simulink model "gm_fft_overlap_tomori"  (R2023b)
settings: Solver=VariableStepAuto  StartTime=0.0  StopTime=inf  RelTol=1e-3
InitFcn:
  | fftparrallelout
  | load('dataram.mat')
  | s= fi(exp(-1j*2*pi.*(0:63)/64),1,16,15);
  | fixed_point = fixdt(1,27,20);
  | fixed_pointu = fixdt(0,29,20);
  | fixed = fixdt(1,22,15);
  | const = fixdt(1,18,17);
  | addConst = fixdt(1,18,16);
  | f =10.4e6;
  | f1=45e6;
  | alpha1 =5;
  | beta1 = 0.00001 ;
  | beta2 = 0.99999 ;
  | beta3 = 23;
undefined symbols (not defined in the file or in its folder): j
libraries: dspxfrm3 x11, commrflib2 x4
(part 6 of 10)

== system gm_fft_overlap_tomori/16//32 and test junk/32/FFT32/FFT16/FFT8 ==
  In1 : Inport
  In2 : Inport  Port=2
  In3 : Inport  Port=3
  In4 : Inport  Port=4
  In5 : Inport  Port=5
  In6 : Inport  Port=6
  In7 : Inport  Port=7
  In8 : Inport  Port=8
  Add{,2,4,6,8,10,12,14,16,18,20,22} (12 alike) : Sum  OutDataTypeStr=fixed  RndMeth=Round
  Add{1,3,5,7,9,11,13,15,17,19,21,23} (12 alike) : Sum  Inputs=+-  OutDataTypeStr=fixed  RndMeth=Round
  Delay{,1,4..9,12..13,16..23} (18 alike) : Delay  DelayLength=1
  Delay{2..3,10..11,14..15} (6 alike) : Delay  DelayLength=3
  multByExp(-j*Pi/4) : Subsystem
  multByExp(-j*Pi/4)1 : Subsystem
  multByMinusJ : Subsystem
  multByMinusJ1 : Subsystem
  multByMinusJ2 : Subsystem
  multByMinusJ3 : Subsystem
  x0 : Outport
  x1 : Outport  Port=2  VectorParamsAs1DForOutWhenUnconnected=off
  x2 : Outport  Port=3  VectorParamsAs1DForOutWhenUnconnected=off
  x3 : Outport  Port=4  VectorParamsAs1DForOutWhenUnconnected=off
  x4 : Outport  Port=5  VectorParamsAs1DForOutWhenUnconnected=off
  x5 : Outport  Port=6  VectorParamsAs1DForOutWhenUnconnected=off
  x6 : Outport  Port=7  VectorParamsAs1DForOutWhenUnconnected=off
  x7 : Outport  Port=8  VectorParamsAs1DForOutWhenUnconnected=off
  wires:
  Delay17/1 -> Add21/2, Add20/2
  Delay15/1 -> Add21/1, Add20/1
  Delay23/1 -> x7/1
  Delay22/1 -> x3/1
  Delay21/1 -> x5/1
  Delay20/1 -> x1/1
  multByExp(-j*Pi/4)1/1(Out1) -> multByMinusJ3/1(In1)
  multByExp(-j*Pi/4)/1(Out1) -> Delay16/1
  multByMinusJ3/1(Out1) -> Delay17/1
  Delay16/1 -> Add18/2, Add19/2
  Delay14/1 -> Add19/1, Add18/1
  Add21/1 -> Delay23/1
  Add20/1 -> Delay22/1
  Add19/1 -> Delay21/1
  Add18/1 -> Delay20/1
  Delay19/1 -> x6/1
  Delay18/1 -> x2/1
  Delay11/1 -> Add12/2, Add13/2
  multByMinusJ2/1(Out1) -> Delay11/1
  Add13/1 -> Delay19/1
  Add12/1 -> Delay18/1
  Delay3/1 -> Add12/1, Add13/1
  Add17/1 -> multByExp(-j*Pi/4)1/1(In1)
  Add16/1 -> multByExp(-j*Pi/4)/1(In1)
  Delay9/1 -> Add16/2, Add17/2
  Delay5/1 -> Add16/1, Add17/1
  multByMinusJ1/1(Out1) -> Delay9/1
  multByMinusJ/1(Out1) -> Delay7/1
  Add15/1 -> Delay15/1
  Add14/1 -> Delay14/1
  Delay7/1 -> Add15/2, Add14/2
  Delay1/1 -> Add15/1, Add14/1
  Delay13/1 -> x4/1
  Delay12/1 -> x0/1
  Add23/1 -> Delay13/1
  Add22/1 -> Delay12/1
  Delay10/1 -> Add22/2, Add23/2
  Delay2/1 -> Add23/1, Add22/1
  Delay6/1 -> Add3/2, Add2/2
  Add11/1 -> multByMinusJ2/1(In1)
  Add10/1 -> Delay10/1
  Delay8/1 -> Add10/2, Add11/2
  Delay4/1 -> Add11/1, Add10/1
  Add9/1 -> multByMinusJ1/1(In1)
  Add8/1 -> Delay8/1
  Add7/1 -> multByMinusJ/1(In1)
  Add6/1 -> Delay6/1
  Add5/1 -> Delay5/1
  Add4/1 -> Delay4/1
  In8/1 -> Add9/2, Add8/2
  In4/1 -> Add8/1, Add9/1
  In6/1 -> Add5/2, Add4/2
  In2/1 -> Add4/1, Add5/1
  In7/1 -> Add7/2, Add6/2
  In3/1 -> Add6/1, Add7/1
  Add3/1 -> Delay3/1
  Add2/1 -> Delay2/1
  Delay/1 -> Add3/1, Add2/1
  Add1/1 -> Delay1/1
  Add/1 -> Delay/1
  In5/1 -> Add1/2, Add/2
  In1/1 -> Add/1, Add1/1

== system gm_fft_overlap_tomori/16//32 and test junk/32/FFT32/FFT16/FFT8_1 ==
  In1 : Inport
  In2 : Inport  Port=2
  In3 : Inport  Port=3
  In4 : Inport  Port=4
  In5 : Inport  Port=5
  In6 : Inport  Port=6
  In7 : Inport  Port=7
  In8 : Inport  Port=8
  Add{,2,4,6,8,10,12,14,16,18,20,22} (12 alike) : Sum  OutDataTypeStr=fixed  RndMeth=Round
  Add{1,3,5,7,9,11,13,15,17,19,21,23} (12 alike) : Sum  Inputs=+-  OutDataTypeStr=fixed  RndMeth=Round
  Delay{,1,4..9,12..13,16..23} (18 alike) : Delay  DelayLength=1
  Delay{2..3,10..11,14..15} (6 alike) : Delay  DelayLength=3
  multByExp(-j*Pi/4) : Subsystem
  multByExp(-j*Pi/4)1 : Subsystem
  multByMinusJ : Subsystem
  multByMinusJ1 : Subsystem
  multByMinusJ2 : Subsystem
  multByMinusJ3 : Subsystem
  x0 : Outport
  x1 : Outport  Port=2  VectorParamsAs1DForOutWhenUnconnected=off
  x2 : Outport  Port=3  VectorParamsAs1DForOutWhenUnconnected=off
  x3 : Outport  Port=4  VectorParamsAs1DForOutWhenUnconnected=off
  x4 : Outport  Port=5  VectorParamsAs1DForOutWhenUnconnected=off
  x5 : Outport  Port=6  VectorParamsAs1DForOutWhenUnconnected=off
  x6 : Outport  Port=7  VectorParamsAs1DForOutWhenUnconnected=off
  x7 : Outport  Port=8  VectorParamsAs1DForOutWhenUnconnected=off
  wires:
  Delay17/1 -> Add21/2, Add20/2
  Delay15/1 -> Add21/1, Add20/1
  Delay23/1 -> x7/1
  Delay22/1 -> x3/1
  Delay21/1 -> x5/1
  Delay20/1 -> x1/1
  multByExp(-j*Pi/4)1/1(Out1) -> multByMinusJ3/1(In1)
  multByExp(-j*Pi/4)/1(Out1) -> Delay16/1
  multByMinusJ3/1(Out1) -> Delay17/1
  Delay16/1 -> Add18/2, Add19/2
  Delay14/1 -> Add19/1, Add18/1
  Add21/1 -> Delay23/1
  Add20/1 -> Delay22/1
  Add19/1 -> Delay21/1
  Add18/1 -> Delay20/1
  Delay19/1 -> x6/1
  Delay18/1 -> x2/1
  Delay11/1 -> Add12/2, Add13/2
  multByMinusJ2/1(Out1) -> Delay11/1
  Add13/1 -> Delay19/1
  Add12/1 -> Delay18/1
  Delay3/1 -> Add12/1, Add13/1
  Add17/1 -> multByExp(-j*Pi/4)1/1(In1)
  Add16/1 -> multByExp(-j*Pi/4)/1(In1)
  Delay9/1 -> Add16/2, Add17/2
  Delay5/1 -> Add16/1, Add17/1
  multByMinusJ1/1(Out1) -> Delay9/1
  multByMinusJ/1(Out1) -> Delay7/1
  Add15/1 -> Delay15/1
  Add14/1 -> Delay14/1
  Delay7/1 -> Add15/2, Add14/2
  Delay1/1 -> Add15/1, Add14/1
  Delay13/1 -> x4/1
  Delay12/1 -> x0/1
  Add23/1 -> Delay13/1
  Add22/1 -> Delay12/1
  Delay10/1 -> Add22/2, Add23/2
  Delay2/1 -> Add23/1, Add22/1
  Delay6/1 -> Add3/2, Add2/2
  Add11/1 -> multByMinusJ2/1(In1)
  Add10/1 -> Delay10/1
  Delay8/1 -> Add10/2, Add11/2
  Delay4/1 -> Add11/1, Add10/1
  Add9/1 -> multByMinusJ1/1(In1)
  Add8/1 -> Delay8/1
  Add7/1 -> multByMinusJ/1(In1)
  Add6/1 -> Delay6/1
  Add5/1 -> Delay5/1
  Add4/1 -> Delay4/1
  In8/1 -> Add9/2, Add8/2
  In4/1 -> Add8/1, Add9/1
  In6/1 -> Add5/2, Add4/2
  In2/1 -> Add4/1, Add5/1
  In7/1 -> Add7/2, Add6/2
  In3/1 -> Add6/1, Add7/1
  Add3/1 -> Delay3/1
  Add2/1 -> Delay2/1
  Delay/1 -> Add3/1, Add2/1
  Add1/1 -> Delay1/1
  Add/1 -> Delay/1
  In5/1 -> Add1/2, Add/2
  In1/1 -> Add/1, Add1/1

== system gm_fft_overlap_tomori/16//32 and test junk/32/FFT32/FFT16/complexmult ==
  x1 : Inport
  In3 : Inport  Port=2
  Add1 : Sum  OutDataTypeStr=fixed  RndMeth=Round
  Add20 : Sum  OutDataTypeStr=fixed  RndMeth=Round
  Add3 : Sum  Inputs=+--  OutDataTypeStr=fixed  AccumDataTypeStr=fixed  RndMeth=Round
  Add4 : Sum  Inputs=+-  OutDataTypeStr=fixed  AccumDataTypeStr=fixed  RndMeth=Round
  Complex to Real-Imag : ComplexToRealImag
  Complex to Real-Imag1 : ComplexToRealImag
  Constant : Constant  Commented=on  Value=1+j  OutDataTypeStr=fixdt(1,22, 15)  SampleTime=2e-8
  Constant1 : Constant  Commented=on  Value=1-j  OutDataTypeStr=fixdt(1,22, 15)  SampleTime=2e-8
  Delay : Delay  DelayLength=3
  Delay1 : Delay  DelayLength=3
  Delay2 : Delay  DelayLength=3
  Display : Display  Commented=on
  Product : Product  OutDataTypeStr=fixed  RndMeth=Round
  Product1 : Product  OutDataTypeStr=fixed  RndMeth=Round
  Product2 : Product  OutDataTypeStr=fixed  RndMeth=Round
  Real-Imag to Complex : RealImagToComplex
  Out1 : Outport
  wires:
  Real-Imag to Complex/1 -> Out1/1
  In3/1 -> Complex to Real-Imag1/1
  x1/1 -> Complex to Real-Imag/1
  Product/1 -> Delay/1
  Product1/1 -> Delay1/1
  Product2/1 -> Delay2/1
  Delay/1 -> Add3/1
  Delay1/1 -> Add4/1, Add3/2
  Delay2/1 -> Add3/3, Add4/2
  Add4/1 -> Real-Imag to Complex/1
  Add3/1 -> Real-Imag to Complex/2
  Add20/1 -> Product/1
  Add1/1 -> Product/2
  Complex to Real-Imag/1 -> Product1/1, Add20/1
  Complex to Real-Imag1/1 -> Product1/2, Add1/1
  Complex to Real-Imag/2 -> Product2/1, Add20/2
  Complex to Real-Imag1/2 -> Product2/2, Add1/2

== system gm_fft_overlap_tomori/16//32 and test junk/32/FFT32/FFT16/complexmult1 ==
  x1 : Inport
  In3 : Inport  Port=2
  Add1 : Sum  OutDataTypeStr=fixed  RndMeth=Round
  Add20 : Sum  OutDataTypeStr=fixed  RndMeth=Round
  Add3 : Sum  Inputs=+--  OutDataTypeStr=fixed  AccumDataTypeStr=fixed  RndMeth=Round
  Add4 : Sum  Inputs=+-  OutDataTypeStr=fixed  AccumDataTypeStr=fixed  RndMeth=Round
  Complex to Real-Imag : ComplexToRealImag
  Complex to Real-Imag1 : ComplexToRealImag
  Constant : Constant  Commented=on  Value=1+j  OutDataTypeStr=fixdt(1,22, 15)  SampleTime=2e-8
  Constant1 : Constant  Commented=on  Value=1-j  OutDataTypeStr=fixdt(1,22, 15)  SampleTime=2e-8
  Delay : Delay  DelayLength=3
  Delay1 : Delay  DelayLength=3
  Delay2 : Delay  DelayLength=3
  Display : Display  Commented=on
  Product : Product  OutDataTypeStr=fixed  RndMeth=Round
  Product1 : Product  OutDataTypeStr=fixed  RndMeth=Round
  Product2 : Product  OutDataTypeStr=fixed  RndMeth=Round
  Real-Imag to Complex : RealImagToComplex
  Out1 : Outport
  wires:
  Complex to Real-Imag1/2 -> Add1/2, Product2/2
  Complex to Real-Imag/2 -> Add20/2, Product2/1
  Complex to Real-Imag1/1 -> Add1/1, Product1/2
  Complex to Real-Imag/1 -> Add20/1, Product1/1
  Add1/1 -> Product/2
  Add20/1 -> Product/1
  Add3/1 -> Real-Imag to Complex/2
  Add4/1 -> Real-Imag to Complex/1
  Delay2/1 -> Add4/2, Add3/3
  Delay1/1 -> Add3/2, Add4/1
  Delay/1 -> Add3/1
  Product2/1 -> Delay2/1
  Product1/1 -> Delay1/1
  Product/1 -> Delay/1
  x1/1 -> Complex to Real-Imag/1
  In3/1 -> Complex to Real-Imag1/1
  Real-Imag to Complex/1 -> Out1/1

== system gm_fft_overlap_tomori/16//32 and test junk/32/FFT32/FFT16/complexmult2 ==
  x1 : Inport
  In3 : Inport  Port=2
  Add1 : Sum  OutDataTypeStr=fixed  RndMeth=Round
  Add20 : Sum  OutDataTypeStr=fixed  RndMeth=Round
  Add3 : Sum  Inputs=+--  OutDataTypeStr=fixed  AccumDataTypeStr=fixed  RndMeth=Round
  Add4 : Sum  Inputs=+-  OutDataTypeStr=fixed  AccumDataTypeStr=fixed  RndMeth=Round
  Complex to Real-Imag : ComplexToRealImag
  Complex to Real-Imag1 : ComplexToRealImag
  Constant : Constant  Commented=on  Value=1+j  OutDataTypeStr=fixdt(1,22, 15)  SampleTime=2e-8
  Constant1 : Constant  Commented=on  Value=1-j  OutDataTypeStr=fixdt(1,22, 15)  SampleTime=2e-8
  Delay : Delay  DelayLength=3
  Delay1 : Delay  DelayLength=3
  Delay2 : Delay  DelayLength=3
  Display : Display  Commented=on
  Product : Product  OutDataTypeStr=fixed  RndMeth=Round
  Product1 : Product  OutDataTypeStr=fixed  RndMeth=Round
  Product2 : Product  OutDataTypeStr=fixed  RndMeth=Round
  Real-Imag to Complex : RealImagToComplex
  Out1 : Outport
  wires:
  Real-Imag to Complex/1 -> Out1/1
  In3/1 -> Complex to Real-Imag1/1
  x1/1 -> Complex to Real-Imag/1
  Product/1 -> Delay/1
  Product1/1 -> Delay1/1
  Product2/1 -> Delay2/1
  Delay/1 -> Add3/1
  Delay1/1 -> Add4/1, Add3/2
  Delay2/1 -> Add3/3, Add4/2
  Add4/1 -> Real-Imag to Complex/1
  Add3/1 -> Real-Imag to Complex/2
  Add20/1 -> Product/1
  Add1/1 -> Product/2
  Complex to Real-Imag/1 -> Product1/1, Add20/1
  Complex to Real-Imag1/1 -> Product1/2, Add1/1
  Complex to Real-Imag/2 -> Product2/1, Add20/2
  Complex to Real-Imag1/2 -> Product2/2, Add1/2

== system gm_fft_overlap_tomori/16//32 and test junk/32/FFT32/FFT16/complexmult3 ==
  x1 : Inport
  In3 : Inport  Port=2
  Add1 : Sum  OutDataTypeStr=fixed  RndMeth=Round
  Add20 : Sum  OutDataTypeStr=fixed  RndMeth=Round
  Add3 : Sum  Inputs=+--  OutDataTypeStr=fixed  AccumDataTypeStr=fixed  RndMeth=Round
  Add4 : Sum  Inputs=+-  OutDataTypeStr=fixed  AccumDataTypeStr=fixed  RndMeth=Round
  Complex to Real-Imag : ComplexToRealImag
  Complex to Real-Imag1 : ComplexToRealImag
  Constant : Constant  Commented=on  Value=1+j  OutDataTypeStr=fixdt(1,22, 15)  SampleTime=2e-8
  Constant1 : Constant  Commented=on  Value=1-j  OutDataTypeStr=fixdt(1,22, 15)  SampleTime=2e-8
  Delay : Delay  DelayLength=3
  Delay1 : Delay  DelayLength=3
  Delay2 : Delay  DelayLength=3
  Display : Display  Commented=on
  Product : Product  OutDataTypeStr=fixed  RndMeth=Round
  Product1 : Product  OutDataTypeStr=fixed  RndMeth=Round
  Product2 : Product  OutDataTypeStr=fixed  RndMeth=Round
  Real-Imag to Complex : RealImagToComplex
  Out1 : Outport
  wires:
  Complex to Real-Imag1/2 -> Add1/2, Product2/2
  Complex to Real-Imag/2 -> Add20/2, Product2/1
  Complex to Real-Imag1/1 -> Add1/1, Product1/2
  Complex to Real-Imag/1 -> Add20/1, Product1/1
  Add1/1 -> Product/2
  Add20/1 -> Product/1
  Add3/1 -> Real-Imag to Complex/2
  Add4/1 -> Real-Imag to Complex/1
  Delay2/1 -> Add4/2, Add3/3
  Delay1/1 -> Add3/2, Add4/1
  Delay/1 -> Add3/1
  Product2/1 -> Delay2/1
  Product1/1 -> Delay1/1
  Product/1 -> Delay/1
  x1/1 -> Complex to Real-Imag/1
  In3/1 -> Complex to Real-Imag1/1
  Real-Imag to Complex/1 -> Out1/1

== system gm_fft_overlap_tomori/16//32 and test junk/32/FFT32/FFT16/multByExp(-j*Pi//4) ==
  In1 : Inport
  Add : Sum  OutDataTypeStr=fixed  RndMeth=Round
  Add1 : Sum  Inputs=+-  OutDataTypeStr=fixed  RndMeth=Round
  Complex to Real-Imag : ComplexToRealImag
  Delay24 : Delay
  Gain : Gain  Gain=sqrt(2)/2  ParamDataTypeStr=fixed  OutDataTypeStr=fixed  RndMeth=Round
  Real-Imag to Complex : RealImagToComplex
  Out1 : Outport
  wires:
  In1/1 -> Gain/1
  Real-Imag to Complex/1 -> Out1/1
  Delay24/1 -> Complex to Real-Imag/1
  Add1/1 -> Real-Imag to Complex/2
  Add/1 -> Real-Imag to Complex/1
  Complex to Real-Imag/2 -> Add/2, Add1/1
  Complex to Real-Imag/1 -> Add/1, Add1/2
  Gain/1 -> Delay24/1

== system gm_fft_overlap_tomori/16//32 and test junk/32/FFT32/FFT16/multByExp(-j*Pi//4)1 ==
  In1 : Inport
  Add : Sum  OutDataTypeStr=fixed  RndMeth=Round
  Add1 : Sum  Inputs=+-  OutDataTypeStr=fixed  RndMeth=Round
  Complex to Real-Imag : ComplexToRealImag
  Delay24 : Delay
  Gain : Gain  Gain=sqrt(2)/2  ParamDataTypeStr=fixed  OutDataTypeStr=fixed  RndMeth=Round
  Real-Imag to Complex : RealImagToComplex
  Out1 : Outport
  wires:
  Gain/1 -> Delay24/1
  Complex to Real-Imag/1 -> Add1/2, Add/1
  Complex to Real-Imag/2 -> Add1/1, Add/2
  Add/1 -> Real-Imag to Complex/1
  Add1/1 -> Real-Imag to Complex/2
  Delay24/1 -> Complex to Real-Imag/1
  Real-Imag to Complex/1 -> Out1/1
  In1/1 -> Gain/1

== system gm_fft_overlap_tomori/16//32 and test junk/32/FFT32/FFT16/multByMinusJ ==
  x4 : Inport
  Complex to Real-Imag : ComplexToRealImag
  Real-Imag to Complex : RealImagToComplex
  Unary Minus1 : UnaryMinus
  Out1 : Outport
  wires:
  Complex to Real-Imag/1 -> Unary Minus1/1
  Complex to Real-Imag/2 -> Real-Imag to Complex/1
  x4/1 -> Complex to Real-Imag/1
  Real-Imag to Complex/1 -> Out1/1
  Unary Minus1/1 -> Real-Imag to Complex/2

== system gm_fft_overlap_tomori/16//32 and test junk/32/FFT32/FFT16/multByMinusJ3 ==
  In1 : Inport
  Complex to Real-Imag : ComplexToRealImag
  Real-Imag to Complex : RealImagToComplex
  Unary Minus1 : UnaryMinus
  Out1 : Outport
  wires:
  Complex to Real-Imag/1 -> Unary Minus1/1
  Complex to Real-Imag/2 -> Real-Imag to Complex/1
  In1/1 -> Complex to Real-Imag/1
  Real-Imag to Complex/1 -> Out1/1
  Unary Minus1/1 -> Real-Imag to Complex/2

== system gm_fft_overlap_tomori/16//32 and test junk/32/FFT32/FFT16/test ==
  In1 : Inport
  Abs1 : Abs  Commented=on  SaturateOnIntegerOverflow=off
  Abs2 : Abs  Commented=on  SaturateOnIntegerOverflow=off
  Buffer1 : Buffer  Commented=on  N=8  V=7  OutputFrames=off
  Data Type Conversion1 : DataTypeConversion  Commented=on  OutDataTypeStr=fixdt(1,16,15)  SaturateOnIntegerOverflow=off  RndMeth=Floor
  Data Type Conversion2 : DataTypeConversion  Commented=on  OutDataTypeStr=fixdt(1,16,15)  SaturateOnIntegerOverflow=off  RndMeth=Floor
  Data Type Conversion4 : DataTypeConversion  Commented=on  OutDataTypeStr=double  SaturateOnIntegerOverflow=off  RndMeth=Floor
  Data Type Conversion5 : DataTypeConversion  Commented=on  OutDataTypeStr=double  SaturateOnIntegerOverflow=off  RndMeth=Floor
  Data Type Conversion6 : DataTypeConversion  Commented=on  SaturateOnIntegerOverflow=off  RndMeth=Floor
  Delay{28..34} (7 alike) : Delay  Commented=on  DelayLength=1
  Delay35 : Delay  Commented=on  DelayLength=40
  FFT1 : dspxfrm3/FFT  Commented=on  FFTImplementation=Auto  CompMethod=Table lookup  TableOpt=NEW  TableOptActive=Speed  BitRevOrder=off  Normalize=off  InheritFFTLength=on  FFTLength=64  WrapInput=on  roundingMode=Floor  overflowMode=off  firstCoeffDataTypeStr=Inherit: Same word length as input  firstCoeffLastDataTypeStr=Inherit: Same word length as input  outputMin=[]  outputMax=[]
  Mux : Mux  Commented=on  Inputs=8
  Real-Imag to Complex : RealImagToComplex  Commented=on
  Real-Imag to Complex1 : RealImagToComplex  Commented=on
  Scope : Scope  Commented=on  NumInputPorts=2
  Scope1 : Scope  NumInputPorts=8
  Sine Wave1 : Sin  Commented=on  Frequency=2*pi*1e6  SampleTime=2e-8
  Sine Wave2 : Sin  Commented=on  Frequency=2*pi*1e6  SampleTime=2e-8
  Sine Wave3 : Sin  Commented=on  Amplitude=.99  Frequency=2*pi*1e6  Phase=pi/2  SampleTime=2e-8
  Sine Wave4 : Sin  Commented=on  Amplitude=.99  Frequency=2*pi*1e6  Phase=pi/2  SampleTime=2e-8
  Unbuffer1 : Unbuffer  Commented=on
  Unbuffer2 : Unbuffer  Commented=on
  Out1 : Outport
  wires:
  Unbuffer2/1 -> Data Type Conversion5/1
  Abs2/1 -> Delay35/1
  Real-Imag to Complex1/1 -> Data Type Conversion1/1
  Sine Wave2/1 -> Real-Imag to Complex/2
  Abs1/1 -> Scope/1
  Buffer1/1 -> FFT1/1
  Delay33/1 -> Delay34/1
  Data Type Conversion6/1 -> Buffer1/1
  Delay35/1 -> Scope/2
  Real-Imag to Complex/1 -> Data Type Conversion2/1
  Sine Wave4/1 -> Real-Imag to Complex1/1
  Delay29/1 -> Delay30/1
  Delay31/1 -> Delay32/1
  Delay28/1 -> Delay29/1
  Sine Wave3/1 -> Real-Imag to Complex/1
  Data Type Conversion4/1 -> Abs1/1
  Data Type Conversion5/1 -> Abs2/1
  Data Type Conversion1/1 -> Delay28/1
  FFT1/1 -> Unbuffer2/1
  Mux/1 -> Unbuffer1/1
  Delay30/1 -> Delay31/1
  Sine Wave1/1 -> Real-Imag to Complex1/2
  Data Type Conversion2/1 -> Data Type Conversion6/1
  Unbuffer1/1 -> Data Type Conversion4/1
  Delay32/1 -> Delay33/1
  In1/1 -> Out1/1

== system gm_fft_overlap_tomori/16//32 and test junk/32/FFT32/FFT16_1/FFT8 ==
  In1 : Inport
  In2 : Inport  Port=2
  In3 : Inport  Port=3
  In4 : Inport  Port=4
  In5 : Inport  Port=5
  In6 : Inport  Port=6
  In7 : Inport  Port=7
  In8 : Inport  Port=8
  Add{,2,4,6,8,10,12,14,16,18,20,22} (12 alike) : Sum  OutDataTypeStr=fixed  RndMeth=Round
  Add{1,3,5,7,9,11,13,15,17,19,21,23} (12 alike) : Sum  Inputs=+-  OutDataTypeStr=fixed  RndMeth=Round
  Delay{,1,4..9,12..13,16..23} (18 alike) : Delay  DelayLength=1
  Delay{2..3,10..11,14..15} (6 alike) : Delay  DelayLength=3
  multByExp(-j*Pi/4) : Subsystem
  multByExp(-j*Pi/4)1 : Subsystem
  multByMinusJ : Subsystem
  multByMinusJ1 : Subsystem
  multByMinusJ2 : Subsystem
  multByMinusJ3 : Subsystem
  x0 : Outport
  x1 : Outport  Port=2  VectorParamsAs1DForOutWhenUnconnected=off
  x2 : Outport  Port=3  VectorParamsAs1DForOutWhenUnconnected=off
  x3 : Outport  Port=4  VectorParamsAs1DForOutWhenUnconnected=off
  x4 : Outport  Port=5  VectorParamsAs1DForOutWhenUnconnected=off
  x5 : Outport  Port=6  VectorParamsAs1DForOutWhenUnconnected=off
  x6 : Outport  Port=7  VectorParamsAs1DForOutWhenUnconnected=off
  x7 : Outport  Port=8  VectorParamsAs1DForOutWhenUnconnected=off
  wires:
  In1/1 -> Add1/1, Add/1
  In5/1 -> Add/2, Add1/2
  Add/1 -> Delay/1
  Add1/1 -> Delay1/1
  Delay/1 -> Add2/1, Add3/1
  Add2/1 -> Delay2/1
  Add3/1 -> Delay3/1
  In3/1 -> Add7/1, Add6/1
  In7/1 -> Add6/2, Add7/2
  In2/1 -> Add5/1, Add4/1
  In6/1 -> Add4/2, Add5/2
  In4/1 -> Add9/1, Add8/1
  In8/1 -> Add8/2, Add9/2
  Add4/1 -> Delay4/1
  Add5/1 -> Delay5/1
  Add6/1 -> Delay6/1
  Add7/1 -> multByMinusJ/1(In1)
  Add8/1 -> Delay8/1
  Add9/1 -> multByMinusJ1/1(In1)
  Delay4/1 -> Add10/1, Add11/1
  Delay8/1 -> Add11/2, Add10/2
  Add10/1 -> Delay10/1
  Add11/1 -> multByMinusJ2/1(In1)
  Delay6/1 -> Add2/2, Add3/2
  Delay2/1 -> Add22/1, Add23/1
  Delay10/1 -> Add23/2, Add22/2
  Add22/1 -> Delay12/1
  Add23/1 -> Delay13/1
  Delay12/1 -> x0/1
  Delay13/1 -> x4/1
  Delay1/1 -> Add14/1, Add15/1
  Delay7/1 -> Add14/2, Add15/2
  Add14/1 -> Delay14/1
  Add15/1 -> Delay15/1
  multByMinusJ/1(Out1) -> Delay7/1
  multByMinusJ1/1(Out1) -> Delay9/1
  Delay5/1 -> Add17/1, Add16/1
  Delay9/1 -> Add17/2, Add16/2
  Add16/1 -> multByExp(-j*Pi/4)/1(In1)
  Add17/1 -> multByExp(-j*Pi/4)1/1(In1)
  Delay3/1 -> Add13/1, Add12/1
  Add12/1 -> Delay18/1
  Add13/1 -> Delay19/1
  multByMinusJ2/1(Out1) -> Delay11/1
  Delay11/1 -> Add13/2, Add12/2
  Delay18/1 -> x2/1
  Delay19/1 -> x6/1
  Add18/1 -> Delay20/1
  Add19/1 -> Delay21/1
  Add20/1 -> Delay22/1
  Add21/1 -> Delay23/1
  Delay14/1 -> Add18/1, Add19/1
  Delay16/1 -> Add19/2, Add18/2
  multByMinusJ3/1(Out1) -> Delay17/1
  multByExp(-j*Pi/4)/1(Out1) -> Delay16/1
  multByExp(-j*Pi/4)1/1(Out1) -> multByMinusJ3/1(In1)
  Delay20/1 -> x1/1
  Delay21/1 -> x5/1
  Delay22/1 -> x3/1
  Delay23/1 -> x7/1
  Delay15/1 -> Add20/1, Add21/1
  Delay17/1 -> Add20/2, Add21/2

== system gm_fft_overlap_tomori/16//32 and test junk/32/FFT32/FFT16_1/FFT8_1 ==
  In1 : Inport
  In2 : Inport  Port=2
  In3 : Inport  Port=3
  In4 : Inport  Port=4
  In5 : Inport  Port=5
  In6 : Inport  Port=6
  In7 : Inport  Port=7
  In8 : Inport  Port=8
  Add{,2,4,6,8,10,12,14,16,18,20,22} (12 alike) : Sum  OutDataTypeStr=fixed  RndMeth=Round
  Add{1,3,5,7,9,11,13,15,17,19,21,23} (12 alike) : Sum  Inputs=+-  OutDataTypeStr=fixed  RndMeth=Round
  Delay{,1,4..9,12..13,16..23} (18 alike) : Delay  DelayLength=1
  Delay{2..3,10..11,14..15} (6 alike) : Delay  DelayLength=3
  multByExp(-j*Pi/4) : Subsystem
  multByExp(-j*Pi/4)1 : Subsystem
  multByMinusJ : Subsystem
  multByMinusJ1 : Subsystem
  multByMinusJ2 : Subsystem
  multByMinusJ3 : Subsystem
  x0 : Outport
  x1 : Outport  Port=2  VectorParamsAs1DForOutWhenUnconnected=off
  x2 : Outport  Port=3  VectorParamsAs1DForOutWhenUnconnected=off
  x3 : Outport  Port=4  VectorParamsAs1DForOutWhenUnconnected=off
  x4 : Outport  Port=5  VectorParamsAs1DForOutWhenUnconnected=off
  x5 : Outport  Port=6  VectorParamsAs1DForOutWhenUnconnected=off
  x6 : Outport  Port=7  VectorParamsAs1DForOutWhenUnconnected=off
  x7 : Outport  Port=8  VectorParamsAs1DForOutWhenUnconnected=off
  wires:
  In1/1 -> Add1/1, Add/1
  In5/1 -> Add/2, Add1/2
  Add/1 -> Delay/1
  Add1/1 -> Delay1/1
  Delay/1 -> Add2/1, Add3/1
  Add2/1 -> Delay2/1
  Add3/1 -> Delay3/1
  In3/1 -> Add7/1, Add6/1
  In7/1 -> Add6/2, Add7/2
  In2/1 -> Add5/1, Add4/1
  In6/1 -> Add4/2, Add5/2
  In4/1 -> Add9/1, Add8/1
  In8/1 -> Add8/2, Add9/2
  Add4/1 -> Delay4/1
  Add5/1 -> Delay5/1
  Add6/1 -> Delay6/1
  Add7/1 -> multByMinusJ/1(In1)
  Add8/1 -> Delay8/1
  Add9/1 -> multByMinusJ1/1(In1)
  Delay4/1 -> Add10/1, Add11/1
  Delay8/1 -> Add11/2, Add10/2
  Add10/1 -> Delay10/1
  Add11/1 -> multByMinusJ2/1(In1)
  Delay6/1 -> Add2/2, Add3/2
  Delay2/1 -> Add22/1, Add23/1
  Delay10/1 -> Add23/2, Add22/2
  Add22/1 -> Delay12/1
  Add23/1 -> Delay13/1
  Delay12/1 -> x0/1
  Delay13/1 -> x4/1
  Delay1/1 -> Add14/1, Add15/1
  Delay7/1 -> Add14/2, Add15/2
  Add14/1 -> Delay14/1
  Add15/1 -> Delay15/1
  multByMinusJ/1(Out1) -> Delay7/1
  multByMinusJ1/1(Out1) -> Delay9/1
  Delay5/1 -> Add17/1, Add16/1
  Delay9/1 -> Add17/2, Add16/2
  Add16/1 -> multByExp(-j*Pi/4)/1(In1)
  Add17/1 -> multByExp(-j*Pi/4)1/1(In1)
  Delay3/1 -> Add13/1, Add12/1
  Add12/1 -> Delay18/1
  Add13/1 -> Delay19/1
  multByMinusJ2/1(Out1) -> Delay11/1
  Delay11/1 -> Add13/2, Add12/2
  Delay18/1 -> x2/1
  Delay19/1 -> x6/1
  Add18/1 -> Delay20/1
  Add19/1 -> Delay21/1
  Add20/1 -> Delay22/1
  Add21/1 -> Delay23/1
  Delay14/1 -> Add18/1, Add19/1
  Delay16/1 -> Add19/2, Add18/2
  multByMinusJ3/1(Out1) -> Delay17/1
  multByExp(-j*Pi/4)/1(Out1) -> Delay16/1
  multByExp(-j*Pi/4)1/1(Out1) -> multByMinusJ3/1(In1)
  Delay20/1 -> x1/1
  Delay21/1 -> x5/1
  Delay22/1 -> x3/1
  Delay23/1 -> x7/1
  Delay15/1 -> Add20/1, Add21/1
  Delay17/1 -> Add20/2, Add21/2

== system gm_fft_overlap_tomori/16//32 and test junk/32/FFT32/FFT16_1/complexmult ==
  x1 : Inport
  In3 : Inport  Port=2
  Add1 : Sum  OutDataTypeStr=fixed  RndMeth=Round
  Add20 : Sum  OutDataTypeStr=fixed  RndMeth=Round
  Add3 : Sum  Inputs=+--  OutDataTypeStr=fixed  AccumDataTypeStr=fixed  RndMeth=Round
  Add4 : Sum  Inputs=+-  OutDataTypeStr=fixed  AccumDataTypeStr=fixed  RndMeth=Round
  Complex to Real-Imag : ComplexToRealImag
  Complex to Real-Imag1 : ComplexToRealImag
  Constant : Constant  Commented=on  Value=1+j  OutDataTypeStr=fixdt(1,22, 15)  SampleTime=2e-8
  Constant1 : Constant  Commented=on  Value=1-j  OutDataTypeStr=fixdt(1,22, 15)  SampleTime=2e-8
  Delay : Delay  DelayLength=3
  Delay1 : Delay  DelayLength=3
  Delay2 : Delay  DelayLength=3
  Display : Display  Commented=on
  Product : Product  OutDataTypeStr=fixed  RndMeth=Round
  Product1 : Product  OutDataTypeStr=fixed  RndMeth=Round
  Product2 : Product  OutDataTypeStr=fixed  RndMeth=Round
  Real-Imag to Complex : RealImagToComplex
  Out1 : Outport
  wires:
  Complex to Real-Imag1/2 -> Add1/2, Product2/2
  Complex to Real-Imag/2 -> Add20/2, Product2/1
  Complex to Real-Imag1/1 -> Add1/1, Product1/2
  Complex to Real-Imag/1 -> Add20/1, Product1/1
  Add1/1 -> Product/2
  Add20/1 -> Product/1
  Add3/1 -> Real-Imag to Complex/2
  Add4/1 -> Real-Imag to Complex/1
  Delay2/1 -> Add4/2, Add3/3
  Delay1/1 -> Add3/2, Add4/1
  Delay/1 -> Add3/1
  Product2/1 -> Delay2/1
  Product1/1 -> Delay1/1
  Product/1 -> Delay/1
  x1/1 -> Complex to Real-Imag/1
  In3/1 -> Complex to Real-Imag1/1
  Real-Imag to Complex/1 -> Out1/1

== system gm_fft_overlap_tomori/16//32 and test junk/32/FFT32/FFT16_1/complexmult1 ==
  x1 : Inport
  In3 : Inport  Port=2
  Add1 : Sum  OutDataTypeStr=fixed  RndMeth=Round
  Add20 : Sum  OutDataTypeStr=fixed  RndMeth=Round
  Add3 : Sum  Inputs=+--  OutDataTypeStr=fixed  AccumDataTypeStr=fixed  RndMeth=Round
  Add4 : Sum  Inputs=+-  OutDataTypeStr=fixed  AccumDataTypeStr=fixed  RndMeth=Round
  Complex to Real-Imag : ComplexToRealImag
  Complex to Real-Imag1 : ComplexToRealImag
  Constant : Constant  Commented=on  Value=1+j  OutDataTypeStr=fixdt(1,22, 15)  SampleTime=2e-8
  Constant1 : Constant  Commented=on  Value=1-j  OutDataTypeStr=fixdt(1,22, 15)  SampleTime=2e-8
  Delay : Delay  DelayLength=3
  Delay1 : Delay  DelayLength=3
  Delay2 : Delay  DelayLength=3
  Display : Display  Commented=on
  Product : Product  OutDataTypeStr=fixed  RndMeth=Round
  Product1 : Product  OutDataTypeStr=fixed  RndMeth=Round
  Product2 : Product  OutDataTypeStr=fixed  RndMeth=Round
  Real-Imag to Complex : RealImagToComplex
  Out1 : Outport
  wires:
  Real-Imag to Complex/1 -> Out1/1
  In3/1 -> Complex to Real-Imag1/1
  x1/1 -> Complex to Real-Imag/1
  Product/1 -> Delay/1
  Product1/1 -> Delay1/1
  Product2/1 -> Delay2/1
  Delay/1 -> Add3/1
  Delay1/1 -> Add4/1, Add3/2
  Delay2/1 -> Add3/3, Add4/2
  Add4/1 -> Real-Imag to Complex/1
  Add3/1 -> Real-Imag to Complex/2
  Add20/1 -> Product/1
  Add1/1 -> Product/2
  Complex to Real-Imag/1 -> Product1/1, Add20/1
  Complex to Real-Imag1/1 -> Product1/2, Add1/1
  Complex to Real-Imag/2 -> Product2/1, Add20/2
  Complex to Real-Imag1/2 -> Product2/2, Add1/2

== system gm_fft_overlap_tomori/16//32 and test junk/32/FFT32/FFT16_1/complexmult2 ==
  x1 : Inport
  In3 : Inport  Port=2
  Add1 : Sum  OutDataTypeStr=fixed  RndMeth=Round
  Add20 : Sum  OutDataTypeStr=fixed  RndMeth=Round
  Add3 : Sum  Inputs=+--  OutDataTypeStr=fixed  AccumDataTypeStr=fixed  RndMeth=Round
  Add4 : Sum  Inputs=+-  OutDataTypeStr=fixed  AccumDataTypeStr=fixed  RndMeth=Round
  Complex to Real-Imag : ComplexToRealImag
  Complex to Real-Imag1 : ComplexToRealImag
  Constant : Constant  Commented=on  Value=1+j  OutDataTypeStr=fixdt(1,22, 15)  SampleTime=2e-8
  Constant1 : Constant  Commented=on  Value=1-j  OutDataTypeStr=fixdt(1,22, 15)  SampleTime=2e-8
  Delay : Delay  DelayLength=3
  Delay1 : Delay  DelayLength=3
  Delay2 : Delay  DelayLength=3
  Display : Display  Commented=on
  Product : Product  OutDataTypeStr=fixed  RndMeth=Round
  Product1 : Product  OutDataTypeStr=fixed  RndMeth=Round
  Product2 : Product  OutDataTypeStr=fixed  RndMeth=Round
  Real-Imag to Complex : RealImagToComplex
  Out1 : Outport
  wires:
  Complex to Real-Imag1/2 -> Add1/2, Product2/2
  Complex to Real-Imag/2 -> Add20/2, Product2/1
  Complex to Real-Imag1/1 -> Add1/1, Product1/2
  Complex to Real-Imag/1 -> Add20/1, Product1/1
  Add1/1 -> Product/2
  Add20/1 -> Product/1
  Add3/1 -> Real-Imag to Complex/2
  Add4/1 -> Real-Imag to Complex/1
  Delay2/1 -> Add4/2, Add3/3
  Delay1/1 -> Add3/2, Add4/1
  Delay/1 -> Add3/1
  Product2/1 -> Delay2/1
  Product1/1 -> Delay1/1
  Product/1 -> Delay/1
  x1/1 -> Complex to Real-Imag/1
  In3/1 -> Complex to Real-Imag1/1
  Real-Imag to Complex/1 -> Out1/1

== system gm_fft_overlap_tomori/16//32 and test junk/32/FFT32/FFT16_1/complexmult3 ==
  x1 : Inport
  In3 : Inport  Port=2
  Add1 : Sum  OutDataTypeStr=fixed  RndMeth=Round
  Add20 : Sum  OutDataTypeStr=fixed  RndMeth=Round
  Add3 : Sum  Inputs=+--  OutDataTypeStr=fixed  AccumDataTypeStr=fixed  RndMeth=Round
  Add4 : Sum  Inputs=+-  OutDataTypeStr=fixed  AccumDataTypeStr=fixed  RndMeth=Round
  Complex to Real-Imag : ComplexToRealImag
  Complex to Real-Imag1 : ComplexToRealImag
  Constant : Constant  Commented=on  Value=1+j  OutDataTypeStr=fixdt(1,22, 15)  SampleTime=2e-8
  Constant1 : Constant  Commented=on  Value=1-j  OutDataTypeStr=fixdt(1,22, 15)  SampleTime=2e-8
  Delay : Delay  DelayLength=3
  Delay1 : Delay  DelayLength=3
  Delay2 : Delay  DelayLength=3
  Display : Display  Commented=on
  Product : Product  OutDataTypeStr=fixed  RndMeth=Round
  Product1 : Product  OutDataTypeStr=fixed  RndMeth=Round
  Product2 : Product  OutDataTypeStr=fixed  RndMeth=Round
  Real-Imag to Complex : RealImagToComplex
  Out1 : Outport
  wires:
  Real-Imag to Complex/1 -> Out1/1
  In3/1 -> Complex to Real-Imag1/1
  x1/1 -> Complex to Real-Imag/1
  Product/1 -> Delay/1
  Product1/1 -> Delay1/1
  Product2/1 -> Delay2/1
  Delay/1 -> Add3/1
  Delay1/1 -> Add4/1, Add3/2
  Delay2/1 -> Add3/3, Add4/2
  Add4/1 -> Real-Imag to Complex/1
  Add3/1 -> Real-Imag to Complex/2
  Add20/1 -> Product/1
  Add1/1 -> Product/2
  Complex to Real-Imag/1 -> Product1/1, Add20/1
  Complex to Real-Imag1/1 -> Product1/2, Add1/1
  Complex to Real-Imag/2 -> Product2/1, Add20/2
  Complex to Real-Imag1/2 -> Product2/2, Add1/2

== system gm_fft_overlap_tomori/16//32 and test junk/32/FFT32/FFT16_1/multByExp(-j*Pi//4) ==
  In1 : Inport
  Add : Sum  OutDataTypeStr=fixed  RndMeth=Round
  Add1 : Sum  Inputs=+-  OutDataTypeStr=fixed  RndMeth=Round
  Complex to Real-Imag : ComplexToRealImag
  Delay24 : Delay
  Gain : Gain  Gain=sqrt(2)/2  ParamDataTypeStr=fixed  OutDataTypeStr=fixed  RndMeth=Round
  Real-Imag to Complex : RealImagToComplex
  Out1 : Outport
  wires:
  Gain/1 -> Delay24/1
  Complex to Real-Imag/1 -> Add1/2, Add/1
  Complex to Real-Imag/2 -> Add1/1, Add/2
  Add/1 -> Real-Imag to Complex/1
  Add1/1 -> Real-Imag to Complex/2
  Delay24/1 -> Complex to Real-Imag/1
  Real-Imag to Complex/1 -> Out1/1
  In1/1 -> Gain/1

== system gm_fft_overlap_tomori/16//32 and test junk/32/FFT32/FFT16_1/multByExp(-j*Pi//4)1 ==
  In1 : Inport
  Add : Sum  OutDataTypeStr=fixed  RndMeth=Round
  Add1 : Sum  Inputs=+-  OutDataTypeStr=fixed  RndMeth=Round
  Complex to Real-Imag : ComplexToRealImag
  Delay24 : Delay
  Gain : Gain  Gain=sqrt(2)/2  ParamDataTypeStr=fixed  OutDataTypeStr=fixed  RndMeth=Round
  Real-Imag to Complex : RealImagToComplex
  Out1 : Outport
  wires:
  In1/1 -> Gain/1
  Real-Imag to Complex/1 -> Out1/1
  Delay24/1 -> Complex to Real-Imag/1
  Add1/1 -> Real-Imag to Complex/2
  Add/1 -> Real-Imag to Complex/1
  Complex to Real-Imag/2 -> Add/2, Add1/1
  Complex to Real-Imag/1 -> Add/1, Add1/2
  Gain/1 -> Delay24/1

== system gm_fft_overlap_tomori/16//32 and test junk/32/FFT32/FFT16_1/multByMinusJ ==
  x4 : Inport
  Complex to Real-Imag : ComplexToRealImag
  Real-Imag to Complex : RealImagToComplex
  Unary Minus1 : UnaryMinus
  Out1 : Outport
  wires:
  Unary Minus1/1 -> Real-Imag to Complex/2
  Real-Imag to Complex/1 -> Out1/1
  x4/1 -> Complex to Real-Imag/1
  Complex to Real-Imag/2 -> Real-Imag to Complex/1
  Complex to Real-Imag/1 -> Unary Minus1/1

== system gm_fft_overlap_tomori/16//32 and test junk/32/FFT32/FFT16_1/multByMinusJ3 ==
  In1 : Inport
  Complex to Real-Imag : ComplexToRealImag
  Real-Imag to Complex : RealImagToComplex
  Unary Minus1 : UnaryMinus
  Out1 : Outport
  wires:
  Unary Minus1/1 -> Real-Imag to Complex/2
  Real-Imag to Complex/1 -> Out1/1
  In1/1 -> Complex to Real-Imag/1
  Complex to Real-Imag/2 -> Real-Imag to Complex/1
  Complex to Real-Imag/1 -> Unary Minus1/1

== system gm_fft_overlap_tomori/16//32 and test junk/32/FFT32/FFT16_1/test ==
  In1 : Inport
  Abs1 : Abs  Commented=on  SaturateOnIntegerOverflow=off
  Abs2 : Abs  Commented=on  SaturateOnIntegerOverflow=off
  Buffer1 : Buffer  Commented=on  N=8  V=7  OutputFrames=off
  Data Type Conversion1 : DataTypeConversion  Commented=on  OutDataTypeStr=fixdt(1,16,15)  SaturateOnIntegerOverflow=off  RndMeth=Floor
  Data Type Conversion2 : DataTypeConversion  Commented=on  OutDataTypeStr=fixdt(1,16,15)  SaturateOnIntegerOverflow=off  RndMeth=Floor
  Data Type Conversion4 : DataTypeConversion  Commented=on  OutDataTypeStr=double  SaturateOnIntegerOverflow=off  RndMeth=Floor
  Data Type Conversion5 : DataTypeConversion  Commented=on  OutDataTypeStr=double  SaturateOnIntegerOverflow=off  RndMeth=Floor
  Data Type Conversion6 : DataTypeConversion  Commented=on  SaturateOnIntegerOverflow=off  RndMeth=Floor
  Delay{28..34} (7 alike) : Delay  Commented=on  DelayLength=1
  Delay35 : Delay  Commented=on  DelayLength=40
  FFT1 : dspxfrm3/FFT  Commented=on  FFTImplementation=Auto  CompMethod=Table lookup  TableOpt=NEW  TableOptActive=Speed  BitRevOrder=off  Normalize=off  InheritFFTLength=on  FFTLength=64  WrapInput=on  roundingMode=Floor  overflowMode=off  firstCoeffDataTypeStr=Inherit: Same word length as input  firstCoeffLastDataTypeStr=Inherit: Same word length as input  outputMin=[]  outputMax=[]
  Mux : Mux  Commented=on  Inputs=8
  Real-Imag to Complex : RealImagToComplex  Commented=on
  Real-Imag to Complex1 : RealImagToComplex  Commented=on
  Scope : Scope  Commented=on  NumInputPorts=2
  Scope1 : Scope  NumInputPorts=8
  Sine Wave1 : Sin  Commented=on  Frequency=2*pi*1e6  SampleTime=2e-8
  Sine Wave2 : Sin  Commented=on  Frequency=2*pi*1e6  SampleTime=2e-8
  Sine Wave3 : Sin  Commented=on  Amplitude=.99  Frequency=2*pi*1e6  Phase=pi/2  SampleTime=2e-8
  Sine Wave4 : Sin  Commented=on  Amplitude=.99  Frequency=2*pi*1e6  Phase=pi/2  SampleTime=2e-8
  Unbuffer1 : Unbuffer  Commented=on
  Unbuffer2 : Unbuffer  Commented=on
  Out1 : Outport
  wires:
  In1/1 -> Out1/1
  Delay32/1 -> Delay33/1
  Unbuffer1/1 -> Data Type Conversion4/1
  Data Type Conversion2/1 -> Data Type Conversion6/1
  Sine Wave1/1 -> Real-Imag to Complex1/2
  Delay30/1 -> Delay31/1
  Mux/1 -> Unbuffer1/1
  FFT1/1 -> Unbuffer2/1
  Data Type Conversion1/1 -> Delay28/1
  Data Type Conversion5/1 -> Abs2/1
  Data Type Conversion4/1 -> Abs1/1
  Sine Wave3/1 -> Real-Imag to Complex/1
  Delay28/1 -> Delay29/1
  Delay31/1 -> Delay32/1
  Delay29/1 -> Delay30/1
  Sine Wave4/1 -> Real-Imag to Complex1/1
  Real-Imag to Complex/1 -> Data Type Conversion2/1
  Delay35/1 -> Scope/2
  Data Type Conversion6/1 -> Buffer1/1
  Delay33/1 -> Delay34/1
  Buffer1/1 -> FFT1/1
  Abs1/1 -> Scope/1
  Sine Wave2/1 -> Real-Imag to Complex/2
  Real-Imag to Complex1/1 -> Data Type Conversion1/1
  Abs2/1 -> Delay35/1
  Unbuffer2/1 -> Data Type Conversion5/1

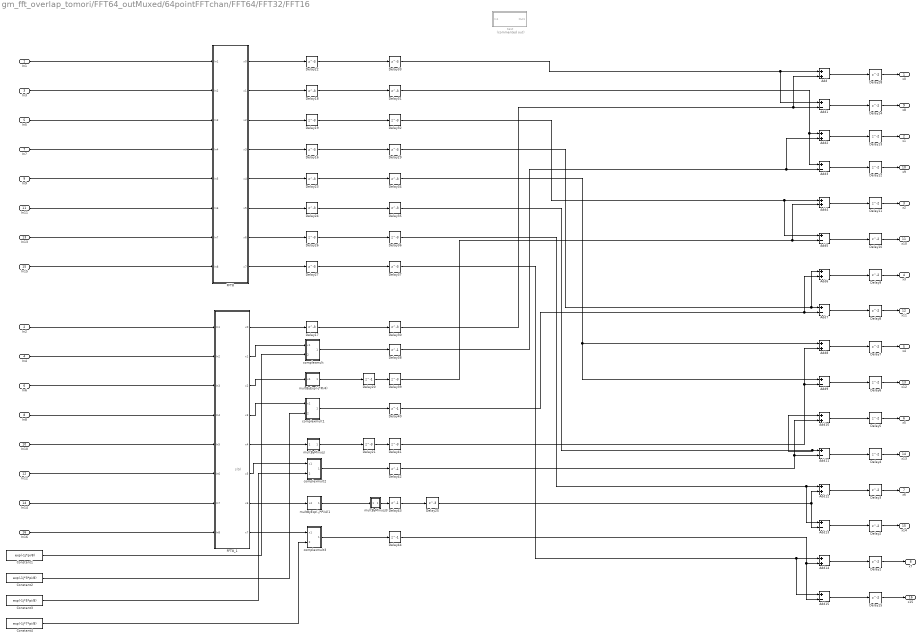
== system gm_fft_overlap_tomori/FFT64_outMuxed/64pointFFTchan/FFT64/FFT32/FFT16 ==
  note: s(5)
  In1 : Inport
  In2 : Inport  Port=2
  In3 : Inport  Port=3
  In4 : Inport  Port=4
  In5 : Inport  Port=5
  In6 : Inport  Port=6
  In7 : Inport  Port=7
  In8 : Inport  Port=8
  In9 : Inport  Port=9
  In10 : Inport  Port=10
  In11 : Inport  Port=11
  In12 : Inport  Port=12
  In13 : Inport  Port=13
  In14 : Inport  Port=14
  In15 : Inport  Port=15
  In16 : Inport  Port=16
  Add{,2,4,6,8,10,12,14} (8 alike) : Sum  OutDataTypeStr=fixed
  Add{1,3,5,7,9,11,13,15} (8 alike) : Sum  Inputs=+-  OutDataTypeStr=fixed
  Constant1 : Constant  Value=exp(-1j*pi/8)  OutDataTypeStr=const  SampleTime=-1
  Constant2 : Constant  Value=exp(-1j*3*pi/8)  OutDataTypeStr=const  SampleTime=-1
  Constant3 : Constant  Value=exp(-1j*5*pi/8)  OutDataTypeStr=const  SampleTime=-1
  Constant4 : Constant  Value=exp(-1j*7*pi/8)  OutDataTypeStr=const  SampleTime=-1
  Delay{1..15,28} (16 alike) : Delay
  Delay{16..19,21..27,29..37,39,41} (22 alike) : Delay  DelayLength=3
  Delay{20,38,40,42..44} (6 alike) : Delay  DelayLength=1
  FFT8 : Subsystem
  FFT8_1 : Subsystem
  complexmult : Subsystem
  complexmult1 : Subsystem
  complexmult2 : Subsystem
  complexmult3 : Subsystem
  multByExp(-j*Pi/4) : Subsystem
  multByExp(-j*Pi/4)1 : Subsystem
  multByMinusJ : Subsystem
  multByMinusJ3 : Subsystem
  test : Subsystem  Commented=on
  x0 : Outport
  x1 : Outport  Port=2
  x2 : Outport  Port=3
  x3 : Outport  Port=4
  x4 : Outport  Port=5
  x5 : Outport  Port=6
  x6 : Outport  Port=7
  x7 : Outport  Port=8
  x8 : Outport  Port=9
  x9 : Outport  Port=10
  x10 : Outport  Port=11
  x11 : Outport  Port=12
  x12 : Outport  Port=13
  x13 : Outport  Port=14
  x14 : Outport  Port=15
  x15 : Outport  Port=16
  wires:
  FFT8_1/1(x0) -> Delay17/1
  Add/1 -> Delay28/1
  Add1/1 -> Delay14/1
  Constant1/1 -> complexmult/2(In3)
  FFT8_1/2(x1) -> complexmult/1(x1)
  FFT8/2(x1) -> Delay18/1
  Add2/1 -> Delay13/1
  complexmult/1(Out1) -> Delay38/1
  Add3/1 -> Delay12/1
  FFT8_1/3(x2) -> multByExp(-j*Pi/4)/1(x4)
  FFT8/3(x2) -> Delay19/1
  Add4/1 -> Delay11/1
  Add5/1 -> Delay10/1
  multByExp(-j*Pi/4)/1(Out1) -> Delay20/1
  Constant2/1 -> complexmult1/2(In3)
  FFT8_1/4(x3) -> complexmult1/1(x1)
  FFT8/4(x3) -> Delay16/1
  complexmult1/1(Out1) -> Delay40/1
  Add6/1 -> Delay9/1
  Add7/1 -> Delay8/1
  FFT8/5(x4) -> Delay23/1
  multByMinusJ/1(Out1) -> Delay21/1
  Add8/1 -> Delay7/1
  Add9/1 -> Delay6/1
  complexmult2/1(Out1) -> Delay42/1
  FFT8/6(x5) -> Delay24/1
  Add10/1 -> Delay5/1
  Add11/1 -> Delay4/1
  Delay28/1 -> x0/1
  Delay13/1 -> x1/1
  Delay11/1 -> x2/1
  Delay9/1 -> x3/1
  Delay7/1 -> x4/1
  Delay5/1 -> x5/1
  Delay14/1 -> x8/1
  Delay12/1 -> x9/1
  Delay10/1 -> x10/1
  Delay8/1 -> x11/1
  Delay6/1 -> x12/1
  Delay4/1 -> x13/1
  Delay3/1 -> x6/1
  Delay1/1 -> x7/1
  Delay2/1 -> x14/1
  Delay15/1 -> x15/1
  FFT8/1(x0) -> Delay22/1
  Delay17/1 -> Delay30/1
  Delay18/1 -> Delay31/1
  Delay20/1 -> Delay39/1
  Delay19/1 -> Delay32/1
  Delay21/1 -> Delay41/1
  FFT8_1/5(x4) -> multByMinusJ/1(x4)
  Delay22/1 -> Delay33/1
  Delay16/1 -> Delay29/1
  Delay23/1 -> Delay34/1
  Delay24/1 -> Delay35/1
  FFT8_1/7(x6) -> multByExp(-j*Pi/4)1/1(x4)
  multByMinusJ3/1(Out1) -> Delay43/1
  FFT8/7(x6) -> Delay26/1
  Delay25/1 -> Add12/2, Add13/2
  Add12/1 -> Delay3/1
  Add13/1 -> Delay2/1
  Constant4/1 -> complexmult3/2(In3)
  FFT8_1/8(x7) -> complexmult3/1(x1)
  complexmult3/1(Out1) -> Delay44/1
  FFT8/8(x7) -> Delay27/1
  Add14/1 -> Delay1/1
  Add15/1 -> Delay15/1
  Delay26/1 -> Delay36/1
  Delay27/1 -> Delay37/1
  FFT8_1/6(x5) -> complexmult2/1(x1)
  Constant3/1 -> complexmult2/2(In3)
  multByExp(-j*Pi/4)1/1(Out1) -> multByMinusJ3/1(In1)
  In1/1 -> FFT8/1(In1)
  In3/1 -> FFT8/2(In2)
  In5/1 -> FFT8/3(In3)
  In7/1 -> FFT8/4(In4)
  In9/1 -> FFT8/5(In5)
  In11/1 -> FFT8/6(In6)
  In13/1 -> FFT8/7(In7)
  In15/1 -> FFT8/8(In8)
  In2/1 -> FFT8_1/1(In1)
  In4/1 -> FFT8_1/2(In2)
  In6/1 -> FFT8_1/3(In3)
  In8/1 -> FFT8_1/4(In4)
  In10/1 -> FFT8_1/5(In5)
  In12/1 -> FFT8_1/6(In6)
  In14/1 -> FFT8_1/7(In7)
  In16/1 -> FFT8_1/8(In8)
  Delay33/1 -> Add1/1, Add/1
  Delay31/1 -> Add3/1, Add2/1
  Delay32/1 -> Add5/1, Add4/1
  Delay29/1 -> Add6/1, Add7/1
  Delay34/1 -> Add9/1, Add8/1
  Delay35/1 -> Add10/1, Add11/1
  Delay36/1 -> Add13/1, Add12/1
  Delay37/1 -> Add15/1, Add14/1
  Delay30/1 -> Add/2, Add1/2
  Delay38/1 -> Add2/2, Add3/2
  Delay39/1 -> Add4/2, Add5/2
  Delay40/1 -> Add6/2, Add7/2
  Delay41/1 -> Add9/2, Add8/2
  Delay42/1 -> Add11/2, Add10/2
  Delay43/1 -> Delay25/1
  Delay44/1 -> Add15/2, Add14/2

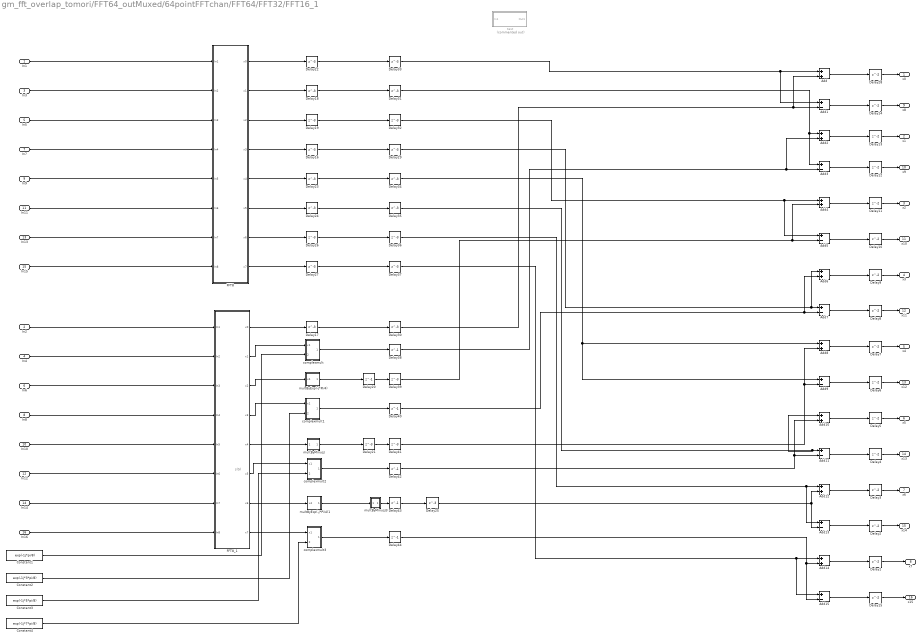
== system gm_fft_overlap_tomori/FFT64_outMuxed/64pointFFTchan/FFT64/FFT32/FFT16_1 ==
  note: s(5)
  In1 : Inport
  In2 : Inport  Port=2
  In3 : Inport  Port=3
  In4 : Inport  Port=4
  In5 : Inport  Port=5
  In6 : Inport  Port=6
  In7 : Inport  Port=7
  In8 : Inport  Port=8
  In9 : Inport  Port=9
  In10 : Inport  Port=10
  In11 : Inport  Port=11
  In12 : Inport  Port=12
  In13 : Inport  Port=13
  In14 : Inport  Port=14
  In15 : Inport  Port=15
  In16 : Inport  Port=16
  Add{,2,4,6,8,10,12,14} (8 alike) : Sum  OutDataTypeStr=fixed
  Add{1,3,5,7,9,11,13,15} (8 alike) : Sum  Inputs=+-  OutDataTypeStr=fixed
  Constant1 : Constant  Value=exp(-1j*pi/8)  OutDataTypeStr=const  SampleTime=-1
  Constant2 : Constant  Value=exp(-1j*3*pi/8)  OutDataTypeStr=const  SampleTime=-1
  Constant3 : Constant  Value=exp(-1j*5*pi/8)  OutDataTypeStr=const  SampleTime=-1
  Constant4 : Constant  Value=exp(-1j*7*pi/8)  OutDataTypeStr=const  SampleTime=-1
  Delay{1..15,28} (16 alike) : Delay
  Delay{16..19,21..27,29..37,39,41} (22 alike) : Delay  DelayLength=3
  Delay{20,38,40,42..44} (6 alike) : Delay  DelayLength=1
  FFT8 : Subsystem
  FFT8_1 : Subsystem
  complexmult : Subsystem
  complexmult1 : Subsystem
  complexmult2 : Subsystem
  complexmult3 : Subsystem
  multByExp(-j*Pi/4) : Subsystem
  multByExp(-j*Pi/4)1 : Subsystem
  multByMinusJ : Subsystem
  multByMinusJ3 : Subsystem
  test : Subsystem  Commented=on
  x0 : Outport
  x1 : Outport  Port=2
  x2 : Outport  Port=3
  x3 : Outport  Port=4
  x4 : Outport  Port=5
  x5 : Outport  Port=6
  x6 : Outport  Port=7
  x7 : Outport  Port=8
  x8 : Outport  Port=9
  x9 : Outport  Port=10
  x10 : Outport  Port=11
  x11 : Outport  Port=12
  x12 : Outport  Port=13
  x13 : Outport  Port=14
  x14 : Outport  Port=15
  x15 : Outport  Port=16
  wires:
  Delay44/1 -> Add14/2, Add15/2
  Delay43/1 -> Delay25/1
  Delay42/1 -> Add10/2, Add11/2
  Delay41/1 -> Add8/2, Add9/2
  Delay40/1 -> Add7/2, Add6/2
  Delay39/1 -> Add5/2, Add4/2
  Delay38/1 -> Add3/2, Add2/2
  Delay30/1 -> Add1/2, Add/2
  Delay37/1 -> Add14/1, Add15/1
  Delay36/1 -> Add12/1, Add13/1
  Delay35/1 -> Add11/1, Add10/1
  Delay34/1 -> Add8/1, Add9/1
  Delay29/1 -> Add7/1, Add6/1
  Delay32/1 -> Add4/1, Add5/1
  Delay31/1 -> Add2/1, Add3/1
  Delay33/1 -> Add/1, Add1/1
  In16/1 -> FFT8_1/8(In8)
  In14/1 -> FFT8_1/7(In7)
  In12/1 -> FFT8_1/6(In6)
  In10/1 -> FFT8_1/5(In5)
  In8/1 -> FFT8_1/4(In4)
  In6/1 -> FFT8_1/3(In3)
  In4/1 -> FFT8_1/2(In2)
  In2/1 -> FFT8_1/1(In1)
  In15/1 -> FFT8/8(In8)
  In13/1 -> FFT8/7(In7)
  In11/1 -> FFT8/6(In6)
  In9/1 -> FFT8/5(In5)
  In7/1 -> FFT8/4(In4)
  In5/1 -> FFT8/3(In3)
  In3/1 -> FFT8/2(In2)
  In1/1 -> FFT8/1(In1)
  multByExp(-j*Pi/4)1/1(Out1) -> multByMinusJ3/1(In1)
  Constant3/1 -> complexmult2/2(In3)
  FFT8_1/6(x5) -> complexmult2/1(x1)
  Delay27/1 -> Delay37/1
  Delay26/1 -> Delay36/1
  Add15/1 -> Delay15/1
  Add14/1 -> Delay1/1
  FFT8/8(x7) -> Delay27/1
  complexmult3/1(Out1) -> Delay44/1
  FFT8_1/8(x7) -> complexmult3/1(x1)
  Constant4/1 -> complexmult3/2(In3)
  Add13/1 -> Delay2/1
  Add12/1 -> Delay3/1
  Delay25/1 -> Add13/2, Add12/2
  FFT8/7(x6) -> Delay26/1
  multByMinusJ3/1(Out1) -> Delay43/1
  FFT8_1/7(x6) -> multByExp(-j*Pi/4)1/1(x4)
  Delay24/1 -> Delay35/1
  Delay23/1 -> Delay34/1
  Delay16/1 -> Delay29/1
  Delay22/1 -> Delay33/1
  FFT8_1/5(x4) -> multByMinusJ/1(x4)
  Delay21/1 -> Delay41/1
  Delay19/1 -> Delay32/1
  Delay20/1 -> Delay39/1
  Delay18/1 -> Delay31/1
  Delay17/1 -> Delay30/1
  FFT8/1(x0) -> Delay22/1
  Delay15/1 -> x15/1
  Delay2/1 -> x14/1
  Delay1/1 -> x7/1
  Delay3/1 -> x6/1
  Delay4/1 -> x13/1
  Delay6/1 -> x12/1
  Delay8/1 -> x11/1
  Delay10/1 -> x10/1
  Delay12/1 -> x9/1
  Delay14/1 -> x8/1
  Delay5/1 -> x5/1
  Delay7/1 -> x4/1
  Delay9/1 -> x3/1
  Delay11/1 -> x2/1
  Delay13/1 -> x1/1
  Delay28/1 -> x0/1
  Add11/1 -> Delay4/1
  Add10/1 -> Delay5/1
  FFT8/6(x5) -> Delay24/1
  complexmult2/1(Out1) -> Delay42/1
  Add9/1 -> Delay6/1
  Add8/1 -> Delay7/1
  multByMinusJ/1(Out1) -> Delay21/1
  FFT8/5(x4) -> Delay23/1
  Add7/1 -> Delay8/1
  Add6/1 -> Delay9/1
  complexmult1/1(Out1) -> Delay40/1
  FFT8/4(x3) -> Delay16/1
  FFT8_1/4(x3) -> complexmult1/1(x1)
  Constant2/1 -> complexmult1/2(In3)
  multByExp(-j*Pi/4)/1(Out1) -> Delay20/1
  Add5/1 -> Delay10/1
  Add4/1 -> Delay11/1
  FFT8/3(x2) -> Delay19/1
  FFT8_1/3(x2) -> multByExp(-j*Pi/4)/1(x4)
  Add3/1 -> Delay12/1
  complexmult/1(Out1) -> Delay38/1
  Add2/1 -> Delay13/1
  FFT8/2(x1) -> Delay18/1
  FFT8_1/2(x1) -> complexmult/1(x1)
  Constant1/1 -> complexmult/2(In3)
  Add1/1 -> Delay14/1
  Add/1 -> Delay28/1
  FFT8_1/1(x0) -> Delay17/1

== system gm_fft_overlap_tomori/FFT64_outMuxed/64pointFFTchan/FFT64/FFT32/complexmult ==
  x1 : Inport
  In3 : Inport  Port=2
  Add1 : Sum  OutDataTypeStr=addConst  RndMeth=Round
  Add2 : Sum  Inputs=+-  OutDataTypeStr=fixed  AccumDataTypeStr=fixed  RndMeth=Round
  Add20 : Sum  OutDataTypeStr=fixed  RndMeth=Round
  Add3 : Sum  Inputs=+-  OutDataTypeStr=fixed  AccumDataTypeStr=fixed  RndMeth=Round
  Add4 : Sum  Inputs=+-  OutDataTypeStr=fixed  AccumDataTypeStr=fixed  RndMeth=Round
  Complex to Real-Imag : ComplexToRealImag
  Complex to Real-Imag1 : ComplexToRealImag
  Constant : Constant  Commented=on  Value=1+j  OutDataTypeStr=fixdt(1,22, 15)  SampleTime=2e-8
  Constant1 : Constant  Commented=on  Value=1-j  OutDataTypeStr=fixdt(1,22, 15)  SampleTime=2e-8
  Data Type Conversion : DataTypeConversion  OutDataTypeStr=fixed  RndMeth=Round  SaturateOnIntegerOverflow=off
  Data Type Conversion1 : DataTypeConversion  OutDataTypeStr=fixed  RndMeth=Round  SaturateOnIntegerOverflow=off
  Data Type Conversion2 : DataTypeConversion  OutDataTypeStr=fixed  RndMeth=Round  SaturateOnIntegerOverflow=off
  Delay : Delay
  Delay1 : Delay
  Delay{3..14} (12 alike) : Delay  DelayLength=1
  Delay2 : Delay
  Display : Display  Commented=on
  Product : Product
  Product1 : Product
  Product2 : Product
  Real-Imag to Complex : RealImagToComplex
  Out1 : Outport
  wires:
  Real-Imag to Complex/1 -> Out1/1
  In3/1 -> Complex to Real-Imag1/1
  x1/1 -> Complex to Real-Imag/1
  Product/1 -> Delay/1
  Product1/1 -> Delay1/1
  Product2/1 -> Delay2/1
  Delay/1 -> Data Type Conversion/1
  Delay1/1 -> Data Type Conversion1/1
  Delay2/1 -> Data Type Conversion2/1
  Add4/1 -> Delay9/1
  Add3/1 -> Delay10/1
  Add20/1 -> Delay3/1
  Add1/1 -> Delay4/1
  Complex to Real-Imag/1 -> Delay5/1, Add20/1
  Complex to Real-Imag1/1 -> Delay6/1, Add1/1
  Complex to Real-Imag/2 -> Delay7/1, Add20/2
  Complex to Real-Imag1/2 -> Delay8/1, Add1/2
  Delay3/1 -> Product/1
  Delay4/1 -> Product/2
  Delay5/1 -> Product1/1
  Delay6/1 -> Product1/2
  Delay7/1 -> Product2/1
  Delay8/1 -> Product2/2
  Delay9/1 -> Real-Imag to Complex/1
  Delay10/1 -> Add2/1
  Delay11/1 -> Add2/2
  Add2/1 -> Real-Imag to Complex/2
  Delay12/1 -> Add3/1
  Data Type Conversion/1 -> Delay12/1
  Data Type Conversion1/1 -> Delay13/1
  Delay13/1 -> Add4/1, Add3/2
  Data Type Conversion2/1 -> Delay14/1
  Delay14/1 -> Delay11/1, Add4/2

== system gm_fft_overlap_tomori/FFT64_outMuxed/64pointFFTchan/FFT64/FFT32/complexmult1 ==
  x1 : Inport
  In3 : Inport  Port=2
  Add1 : Sum  OutDataTypeStr=addConst  RndMeth=Round
  Add2 : Sum  Inputs=+-  OutDataTypeStr=fixed  AccumDataTypeStr=fixed  RndMeth=Round
  Add20 : Sum  OutDataTypeStr=fixed  RndMeth=Round
  Add3 : Sum  Inputs=+-  OutDataTypeStr=fixed  AccumDataTypeStr=fixed  RndMeth=Round
  Add4 : Sum  Inputs=+-  OutDataTypeStr=fixed  AccumDataTypeStr=fixed  RndMeth=Round
  Complex to Real-Imag : ComplexToRealImag
  Complex to Real-Imag1 : ComplexToRealImag
  Constant : Constant  Commented=on  Value=1+j  OutDataTypeStr=fixdt(1,22, 15)  SampleTime=2e-8
  Constant1 : Constant  Commented=on  Value=1-j  OutDataTypeStr=fixdt(1,22, 15)  SampleTime=2e-8
  Data Type Conversion : DataTypeConversion  OutDataTypeStr=fixed  RndMeth=Round  SaturateOnIntegerOverflow=off
  Data Type Conversion1 : DataTypeConversion  OutDataTypeStr=fixed  RndMeth=Round  SaturateOnIntegerOverflow=off
  Data Type Conversion2 : DataTypeConversion  OutDataTypeStr=fixed  RndMeth=Round  SaturateOnIntegerOverflow=off
  Delay : Delay
  Delay1 : Delay
  Delay{3..14} (12 alike) : Delay  DelayLength=1
  Delay2 : Delay
  Display : Display  Commented=on
  Product : Product
  Product1 : Product
  Product2 : Product
  Real-Imag to Complex : RealImagToComplex
  Out1 : Outport
  wires:
  Delay14/1 -> Add4/2, Delay11/1
  Data Type Conversion2/1 -> Delay14/1
  Delay13/1 -> Add3/2, Add4/1
  Data Type Conversion1/1 -> Delay13/1
  Data Type Conversion/1 -> Delay12/1
  Delay12/1 -> Add3/1
  Add2/1 -> Real-Imag to Complex/2
  Delay11/1 -> Add2/2
  Delay10/1 -> Add2/1
  Delay9/1 -> Real-Imag to Complex/1
  Delay8/1 -> Product2/2
  Delay7/1 -> Product2/1
  Delay6/1 -> Product1/2
  Delay5/1 -> Product1/1
  Delay4/1 -> Product/2
  Delay3/1 -> Product/1
  Complex to Real-Imag1/2 -> Add1/2, Delay8/1
  Complex to Real-Imag/2 -> Add20/2, Delay7/1
  Complex to Real-Imag1/1 -> Add1/1, Delay6/1
  Complex to Real-Imag/1 -> Add20/1, Delay5/1
  Add1/1 -> Delay4/1
  Add20/1 -> Delay3/1
  Add3/1 -> Delay10/1
  Add4/1 -> Delay9/1
  Delay2/1 -> Data Type Conversion2/1
  Delay1/1 -> Data Type Conversion1/1
  Delay/1 -> Data Type Conversion/1
  Product2/1 -> Delay2/1
  Product1/1 -> Delay1/1
  Product/1 -> Delay/1
  x1/1 -> Complex to Real-Imag/1
  In3/1 -> Complex to Real-Imag1/1
  Real-Imag to Complex/1 -> Out1/1
